simulink model "Pendulum_Calibration"  (R2024a)
settings: Solver=FixedStepAuto  StartTime=0.0  StopTime=inf  FixedStep=Tc  RelTol=1e-3  EnableMultiTasking=on
libraries: arduinolib x1
settings Model: ExtModeTrigDuration=2  Creator=josep  LastModifiedBy=josep
settings SolverCC: AutoInsertRateTranBlk=on
settings OptimizationCC: EnhancedBackFolding=on  PassReuseOutputArgsAs=Individual arguments  ZeroExternalMemoryAtStartup=off  ZeroInternalMemoryAtStartup=off  MaxStackSize=64  OptimizeBlockOrder=speed  DifferentSizesBufferReuse=on  OptimizationCustomize=off  EfficientTunableParamExpr=on
settings DebuggingCC: ParameterTunabilityLossMsg=error
settings HardwareCC: ProdBitPerInt=16  ProdBitPerPointer=16  ProdBitPerSizeT=16  ProdBitPerPtrDiffT=16  ProdLargestAtomicFloat=None  ProdWordSize=8  ProdHWDeviceType=Atmel->AVR
settings SFSimCC: MATLABDynamicMemAlloc=off
settings RTWCC: Description=Embedded Coder  SystemTargetFile=ert.tlc  HardwareBoard=Arduino Mega 2560  TemplateMakefile=ert_default_tmf  Toolchain=Arduino AVR  BuildConfiguration=Faster Runs
settings CodeAppCC: ForceParamTrailComments=on  IgnoreCustomStorageClasses=off  OperatorAnnotations=on  SimulinkDataObjDesc=on  SFDataObjDesc=on  InsertBlockDesc=on
settings ERTTargetCC: SupportContinuousTime=on  SupportVariableSizeSignals=on  ExtModeTransport=3  ExtModeStaticAlloc=on  ExtModeAutomaticAllocSize=off  ExtModeStaticAllocSize=2048  ExtModeMexFile=ext_xcp  ExtModeIntrfLevel=Level2 - Open

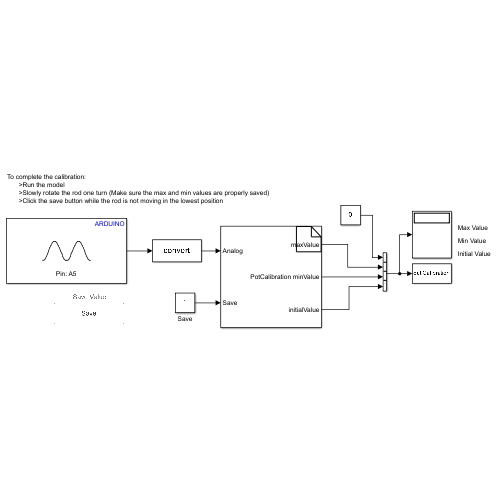
[thumbnail: Simulink's stored preview of the top-level diagram]
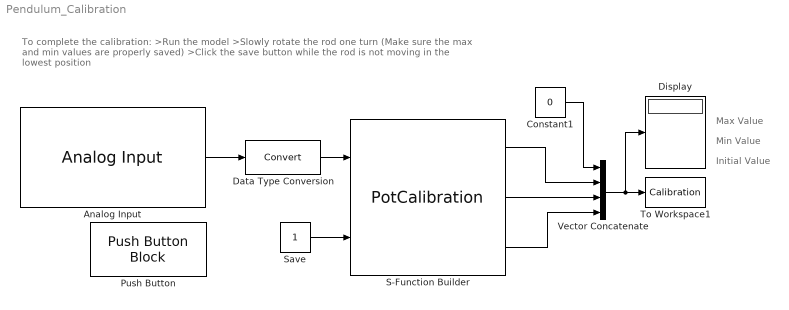
== system Pendulum_Calibration ==
  note: To complete the calibration:
      | >Run the model
      | >Slowly rotate the rod one turn (Make sure the max and min values are properly saved)
      | >Click the save button while the rod is not moving in the lowest position
  note: Min Value
  note: Initial Value
  note: Max Value
  Analog Input : arduinolib/Analog Input  pinNumber=5  ReadResultsOnly=off  ConversionTriggerSource=Software  ExternalTriggerType=uint32( 0 )  OutputDataType=uint16  EnableConversionCompleteNotify=off  EnableOuputStatus=off  SampleTime=-1  blockPlatform=arduino
  Constant1 : Constant  Value=0
  Data Type Conversion : DataTypeConversion  SaturateOnIntegerOverflow=off  RndMeth=Floor
  Display : Display
  Push Button : PushButtonBlock  LabelPosition=Top  ButtonText=Save  OffValue=1.000000
  S-Function Builder : S-Function  InitFcn=try, set_param(gcb,'FunctionName','PotCalibration'), end  FunctionName=PotCalibration  SFunctionModules=PotCalibration_wrapper  SFunctionDeploymentMode=off  EnableBusSupport=off  mask(S-Function Builder){}
      mask help: Simulink:masks:SFunctionBuilder_MD
      mask init:
      | val = [[.9  0.75 0.75 1 1 .9 .9 1]',[1 1 0.75 0.75 .9 .9 1 .9]'];try , sys = get_param(gcb,'SfunBuilderFcnName');if isempty(sys), sys = get_param(gcb,'FunctionName'); end,catch, sys = get_param(gcb,'FunctionName'); end
      settings: CopyFcn=set_param(gcbh,'LinkStatus','none')  PreSaveFcn=try, set_param(gcb,'FunctionName','PotCalibration'), end  OpenFcn=sfunctionwizard(gcbh)
      mask Display: plot(val(:,1),val(:,2)),disp(sys), port_label('input',1,'Analog'), port_label('input',2,'Save'), port_label('output',1,'maxValue'), port_label('output',2,'minValue'), port_label('output',3,'initialValue')
  Save : Constant
  To Workspace1 : ToWorkspace  VariableName=Calibration  SampleTime=-1
      settings: MaxDataPoints=1
  Vector Concatenate : Concatenate  NumInputs=4
  wires:
  S-Function Builder/3 -> Vector Concatenate/4
  Save/1 -> S-Function Builder/2
  Vector Concatenate/1 -> Display/1, To Workspace1/1
  S-Function Builder/1 -> Vector Concatenate/2
  Data Type Conversion/1 -> S-Function Builder/1
  Analog Input/1 -> Data Type Conversion/1
  Constant1/1 -> Vector Concatenate/1
  S-Function Builder/2 -> Vector Concatenate/3
